simulink model "hw3_1a_HillCE"  (R2013a)
settings: Solver=ode45  StartTime=0.0  StopTime=runtime  MaxStep=0.01  RelTol=1e-3
InitFcn:
  | % f-L relationship
  | lopt = 0.08;
  | w = 0.56*lopt;
  | 
  | % f-v relationship
  | K = 5;
  | N = 1.5;
  | vmax = -12*lopt; % m/s, typically expressed as a negative number when talking abotu contraction
  | 
  | % max isometric force
  | Fmax = 6000; % N
  | 
  | % reference strain
  | e_ref = w*2;
  | 
  | runtime = 10;
libraries: simulink x2
settings Model: Creator=benshih  LastModifiedBy=benshih

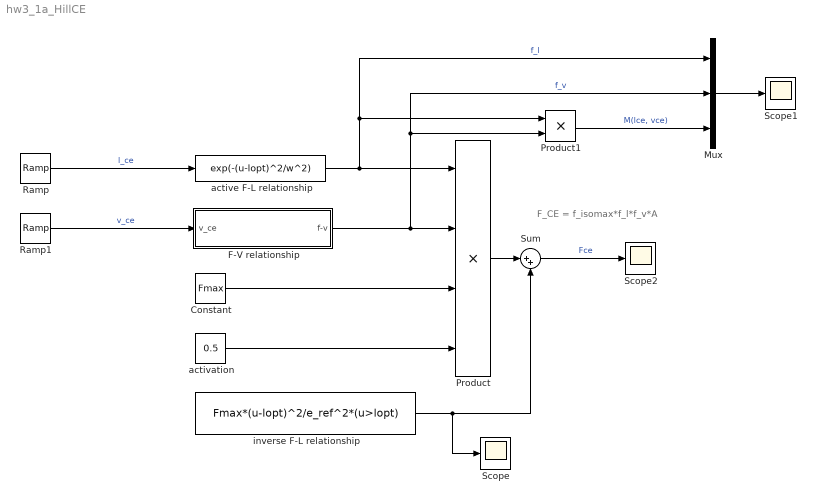
== system hw3_1a_HillCE ==
  note: F_CE = f_isomax*f_l*f_v*A
  Constant : Constant  Value=Fmax
  F-V relationship : Subsystem
  Mux : Mux  Inputs=3
  Product : Product  Inputs=4
  Product1 : Product
  Ramp : simulink/Sources/Ramp  slope=2*lopt/runtime  start=0  X0=0
  Ramp1 : simulink/Sources/Ramp  slope=-vmax*2/runtime  start=0  X0=vmax
  Scope : Scope
  Scope1 : Scope
      settings: SaveName=ScopeData4
  Scope2 : Scope
      settings: SaveName=ScopeData2
  Sum : Sum  Inputs=|++
  activation : Constant  Value=0.5
  active F-L relationship : Fcn  Expr=exp(-(u-lopt)^2/w^2)
  inverse F-L relationship : Fcn  Expr=Fmax*(u-lopt)^2/e_ref^2*(u>lopt)
  wires:
  Ramp/1 -> active F-L relationship/1  "l_ce"
  active F-L relationship/1 -> Mux/1, Product1/1, Product/1  "f_l"
  Ramp1/1 -> F-V relationship/1(v_ce)  "v_ce"
  F-V relationship/1(f-v) -> Mux/2, Product1/2, Product/2  "f_v"
  Constant/1 -> Product/3
  activation/1 -> Product/4
  Product/1 -> Sum/1
  inverse F-L relationship/1 -> Scope/1, Sum/2
  Sum/1 -> Scope2/1  "Fce"
  Product1/1 -> Mux/3  "M(lce, vce)"
  Mux/1 -> Scope1/1

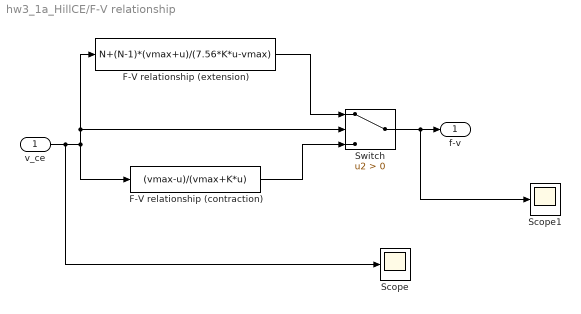
== system hw3_1a_HillCE/F-V relationship ==
  v_ce : Inport
  F-V relationship (contraction) : Fcn  Expr=(vmax-u)/(vmax+K*u)
  F-V relationship (extension) : Fcn  Expr=N+(N-1)*(vmax+u)/(7.56*K*u-vmax)
  Scope : Scope
  Scope1 : Scope
      settings: SaveName=ScopeData3
  Switch : Switch  Criteria=u2 > Threshold
  f-v : Outport
  wires:
  v_ce/1 -> Scope/1, F-V relationship (extension)/1, Switch/2, F-V relationship (contraction)/1
  Switch/1 -> Scope1/1, f-v/1
  F-V relationship (extension)/1 -> Switch/1
  F-V relationship (contraction)/1 -> Switch/3
